simulink model "lb544_rtlsdr_rx_am_ssb_demod"  (R2018b)
settings: Solver=VariableStepAuto  StartTime=0.0  StopTime=inf  RelTol=1e-3
undefined symbols (not defined in the file or in its folder): dfilt, fdesignblkfcn, gcbh
libraries: dspsrcs4 x2, dspsnks4 x1, dspmlti4 x1, dsparch4 x1, sdrrlib x1
settings Model: SimulationMode=accelerator  Creator=Григорий Фокин  LastModifiedBy=Григорий Фокин
settings SFSimCC: SimUseLocalCustomCode=off
settings RTWCC: RTWUseLocalCustomCode=off
settings CodeAppCC: StateflowObjectComments=on

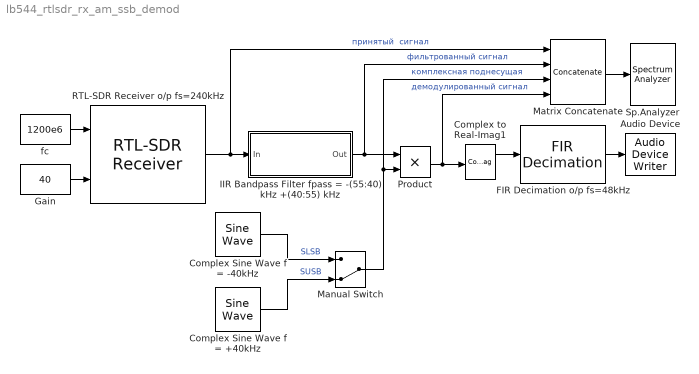
== system lb544_rtlsdr_rx_am_ssb_demod ==
  Audio Device : dspsnks4/Audio Device Writer  Driver=DirectSound  Device=Default  InheritSampleRate=on  SampleRate=44100  BitDepth=16-bit integer  BufferSize=4096  NumBuffers=10  DefaultOutputChannelMapping=on  OutputChannelMapping=1:2  OutputNumUnderrunSamples=off  DriverIdx=1  DeviceWarnFlag=''
  Complex Sine Wave f = +40kHz : dspsrcs4/Sine Wave  Amplitude=1  Frequency=40e3  Phase=0  SampleMode=Discrete  OutComplex=Complex  CompMethod=Trigonometric fcn  TableSize=Speed  SampleTime=1/240e3  SamplesPerFrame=4096  ResetState=Restart at time zero  OutputFrames=on  dataType=single  wordLen=16  udDataType=sfix(16)  fracBitsMode=Best precision  numFracBits=15  OutDataTypeStr=single  LastOutDataTypeStr=single
  Complex Sine Wave f = -40kHz : dspsrcs4/Sine Wave  Amplitude=1  Frequency=-40e3  Phase=0  SampleMode=Discrete  OutComplex=Complex  CompMethod=Trigonometric fcn  TableSize=Speed  SampleTime=1/240e3  SamplesPerFrame=4096  ResetState=Restart at time zero  OutputFrames=on  dataType=single  wordLen=16  udDataType=sfix(16)  fracBitsMode=Best precision  numFracBits=15  OutDataTypeStr=single  LastOutDataTypeStr=single
  Complex to Real-Imag1 : ComplexToRealImag
  FIR Decimation o/p fs=48kHz : dspmlti4/FIR Decimation  FilterSource=Dialog parameters  h=firpm(100, [0 15e3 20e3 (240e3/2)]/(240e3/2), [1 1 0 0], [1 1], 20)  D=5  filtStruct=Direct form  FilterObject=FDECIM  InputProcessing=Columns as channels (frame based)  framing=Allow multirate processing  inputOffset=0  outputBufInitCond=0  roundingMode=Floor  overflowMode=off  firstCoeffDataTypeStr=Inherit: Same word length as input  firstCoeffMin=[]  firstCoeffMax=[]  firstCoeffLastDataTypeStr=Inherit: Same word length as input  outputDataTypeStr=Inherit: Same as accumulator  outputMin=[]  outputMax=[]  outputLastDataTypeStr=Inherit: Same as accumulator
  Gain : Constant  Value=40
  IIR Bandpass Filter fpass = -(55:40) kHz +(40:55) kHz : Subsystem  DialogController=fdesignblkfcn  InitFcn=fdesignblkfcn(gcbh, {'InitFcn'});  mask(Bandpass Filter){}
      mask help: Design a bandpass filter
      settings: CopyFcn=fdesignblkfcn(gcbh, {'CopyFcn'});
      mask Help: helpview(mapfilelocation('dsp'), 'dspbandpassfilter');
      mask Display: disp('Bandpass');
  Manual Switch : ManualSwitch  CurrentSetting=0
  Matrix Concatenate : Concatenate  NumInputs=4  Mode=Multidimensional array  ConcatenateDimension=2
  Product : Product
  RTL-SDR Receiver o/p fs=240kHz : sdrrlib/RTL-SDR Receiver  IPAddress=0  CenterFrequencySource=Input port  CenterFrequency=102.5e6  GainSource=Input port  Gain=0  ADCRate=240e3  FrequencyCorrection=51  LostSamplesOutputPort=off  LatencyOutputPort=off  OutputDataType=single  FrameLength=4096  EnableBurstMode=off  NumFramesInBurst=20  sobjType=sdrr.internal.SDRRTLReceiverSL  dataUDPPort=-1  ctrlUDPPort=-1  subDeviceList=nosubdev  sdrBlockType=SDRBlockTypeSLT.SDRRxBlock  requester=UNUSED_BY_SFCN  sdrExecutionMode=SDRExecutionModeSLT.ExecModeHW  BypassUserLogic=off  DecimatorSelect=DDC decimator  SourceSelect=RF data  SineAmplitude=16000  EnableInternalClock=off  BypassIQBalance=off  IFBandwidth=40e6  ADCRateSource=Dialog  IntermediateFrequency=0  DecimationFactorSource=Dialog  DecimationFactor=512  RFFrequencyIsTunable=logical(1)  SampleTime=(4096)/(240e3)  IFBandwidthSource=Dialog  SineFrequency=30000  BypassDCBlockingFilter=off  IntermediateFrequencySource=Dialog  IQBalanceCoefficients=64  SkipAllHardwareResetAndInitialization=off  EnableIQCalibrationTable=on  CacheIQCalibrationTable=off  EnableOffsetTuning=off  EnableRTLAGC=off  EnableTestMode=off  EnableTunerAGC=off  FrequencyCorrectionSource=Dialog  NumMLBuffers=128  NumUSBBuffers=16  RTLCrystalFrequency=28800000  TunerCrystalFrequency=28800000
      settings: SourceProductName=Communications System Toolbox Support Package for RTL-SDR Radio  SourceProductBaseCode=RTLSDR
  Sp.Analyzer : SpectrumAnalyzer
  fc : Constant  Value=1200e6
  wires:
  fc/1 -> RTL-SDR Receiver o/p fs=240kHz/1
  Gain/1 -> RTL-SDR Receiver o/p fs=240kHz/2
  RTL-SDR Receiver o/p fs=240kHz/1 -> IIR Bandpass Filter fpass = -(55:40) kHz +(40:55) kHz/1(In), Matrix Concatenate/1  "принятый  сигнал"
  IIR Bandpass Filter fpass = -(55:40) kHz +(40:55) kHz/1(Out) -> Product/1, Matrix Concatenate/2  "фильтрованный сигнал"
  Complex to Real-Imag1/1 -> FIR Decimation o/p fs=48kHz/1
  FIR Decimation o/p fs=48kHz/1 -> Audio Device/1
  Matrix Concatenate/1 -> Sp.Analyzer/1
  Product/1 -> Complex to Real-Imag1/1, Matrix Concatenate/4  "демодулированный сигнал"
  Complex Sine Wave f = -40kHz/1 -> Manual Switch/1  "SLSB"
  Complex Sine Wave f = +40kHz/1 -> Manual Switch/2  "SUSB"
  Manual Switch/1 -> Matrix Concatenate/3, Product/2  "комплексная поднесущая"

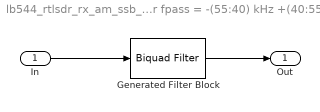
== system lb544_rtlsdr_rx_am_ssb_demod/IIR Bandpass Filter fpass = -(55:40) kHz +(40:55) kHz ==
  In : Inport
  Generated Filter Block : dsparch4/Biquad Filter  Tag=BlockMethodSubSystem  FilterSource=Dialog parameters  CoeffSource=Specify via dialog  FilterObject=dfilt.df2tsos([1 0.3 0.4],[1 0.1 0.2])  IIRFiltStruct=Direct form II  BiQuadCoeffs=[0.42214887875549534 0 -0.42214887875549534 1 -0.98823865611538131 0.97401451420547847;0.033061818692291765 0 -0.033061818692291765 1 -0.255562987775724 0.97029176883907564;0.40962932940897723 0 -0.40962932940897723 1 -0.96374853338649646 0.93400621778983428;0.061627256862270989 0 -0.061627256862270989 1 -0.25549067244038548 0.92491042766383424;0.34804686769186149 0 -0.34804686769186149 1 -0.25882003299069856 0.89279954523166905;0.074485120089956947 0 -0.074485120089956947 1 -0.9294141511065368 0.88695355833419864;0.3380356932077454 0 -0.3380356932077454 1 -0.26749175946597026 0.85279211642514474;0.11414706942811309 0 -0.11414706942811309 1 -0.8993097642364567 0.85187677749258039;0.26975453210172951 0 -0.26975453210172951 1 -0.86713478372906905 0.8192510152074981;0.15169389058649052 0 -0.15169389058649052 1 -0.28068513798157396 0.8162190780957822;0.23486896109857225 0 -0.23486896109857225 1 -0.8331265846567526 0.78923822131355625;0.12543246219034992 0 -0.12543246219034992 1 -0.29806112006699154 0.78328747888967065;0.30344638398123625 0 -0.30344638398123625 1 -0.31363630953671184 0.7610844489222911;0.14204372882356484 0 -0.14204372882356484 1 -0.7883970800288258 0.75566031393796895;0.29204059077048644 0 -0.29204059077048644 1 -0.337525516067535 0.7349293069292292;0.15769964715736565 0 -0.15769964715736565 1 -0.75113712047955783 0.73217586967172454;0.28024335208989254 0 -0.28024335208989254 1 -0.36467175756862613 0.71283395976825903;0.26861034304041859 0 -0.26861034304041859 1 -0.71285267464898394 0.71190933155127689;0.17198129605653537 0 -0.17198129605653537 1 -0.67383770529027076 0.69506646138757555;0.25591667733589984 0 -0.25591667733589984 1 -0.39472573928461274 0.69490448416156714;0.18545503193518079 0 -0.18545503193518079 1 -0.63441698320262108 0.68185149992041572;0.24243607863414046 0 -0.24243607863414046 1 -0.42732343258114791 0.68121939209674687;0.19746276667054932 0 -0.19746276667054932 1 -0.5949462076194667 0.67245728159958573;0.22744846625978013 0 -0.22744846625978013 1 -0.46208364928113799 0.67182458166320957;0.20641989162778182 0 -0.20641989162778182 1 -0.55580817687549611 0.6670545864829549;0.21354369604454937 0 -0.21354369604454937 1 -0.49860880019001874 0.66672790281337901;0.19683387716962003 0 -0.19683387716962003 1 -0.5364892331149077 0.66589493968373292;0.18908777013081096 0 -0.18908777013081096 1 -0.51740549209822551 0.66578232446690089;0.1666062095253458 0 -0.1666062095253458 1 -0.57531079591545409 0.66924746270652935;0.17778848871060463 0 -0.17778848871060463 1 -0.48015100336670025 0.66874010197490674;0.16332726070194734 0 -0.16332726070194734 1 -0.61466449153557434 0.67666548406438465;0.17641184163212795 0 -0.17641184163212795 1 -0.44445772378311499 0.67598426002862111;0.16322683649562625 0 -0.16322683649562625 1 -0.6541565310644416 0.68799304779764836;0.15881803755463447 0 -0.15881803755463447 1 -0.41073003572575306 0.68752769149224158;0.18237880602184384 0 -0.18237880602184384 1 -0.37935764524482984 0.70334288149802093;0.15785452243334397 0 -0.15785452243334397 1 -0.69341695014314575 0.70304702878325664;0.18573995463450585 0 -0.18573995463450585 1 -0.35071303962816736 0.7233669329551885;0.15651735978372061 0 -0.15651735978372061 1 -0.73210527943577131 0.72162757090000862;0.19035218077552934 0 -0.19035218077552934 1 -0.32515241052156241 0.74750700407082749;0.18458592070356522 0 -0.18458592070356522 1 -0.76991241292530632 0.74352854068174234;0.17293280717418719 0 -0.17293280717418719 1 -0.81550826902422946 0.77526501687851923;0.16280924233707353 0 -0.16280924233707353 1 -0.80655855355071004 0.76854651729691692;0.19480307658196594 0 -0.19480307658196594 1 -0.85034522105691646 0.80390751919005965;0.16342802130064965 0 -0.16342802130064965 1 -0.2888713006732021 0.79928652585052429;0.20033951894213034 0 -0.20033951894213034 1 -0.88346607754879403 0.83524758637483043;0.17758411807395799 0 -0.17758411807395799 1 -0.27354455950918161 0.83406249088390871;0.19091925197822526 0 -0.19091925197822526 1 ...(+5184 chars)]  ScaleValues=[0.022496210801432579;1;1;1;1;1;1;1;1;1;1;1;1;1;1;1;1;1;1;1;1;1;1;1;1;1;1;1;1;1;1;1;1;1;1;1;1;1;1;1;1;1;1;1;1;1;1;1;1;1;1;1;1;1;1;1;1;1;1;1;1;1;1;1;1;1;1;1;1;1;1;1;1;1;1;1;1;1;1;1;1;1;1;1;1;1;1;1;1;1;1;1;1;1;1;1;1;1;1;1;1;1;1;1;1;1;1;1]  IC=0  ICnum=0  ICden=0  a0Flag=Warning  optimizeScaleValues=off  ScaleValueMode=Specify via input port (g)  InputProcessing=Columns as channels (frame based)  roundingMode=Floor  overflowMode=off  scaleValueFracLength=14  denProdOutputFracLength=30  denAccumFracLength=30  secondMemoryFracLength=15
      settings: SourceProductName=DSP System Toolbox
  Out : Outport
  wires:
  In/1 -> Generated Filter Block/1
  Generated Filter Block/1 -> Out/1
